simulink library "flexiFlightVis_lib"  (R2018b)
settings: Solver=VariableStepAuto  StartTime=0.0  StopTime=10.0  RelTol=1e-3
values from neighbouring files (symbols this model uses):
  rigid_body = rigidBodyCreate()    [flexiFlightVis_lib_example_init.m]
undefined symbols (not defined in the file or in its folder): config, ffv, ffv_double_array, ffv_double_idx
libraries: dspnetwork x1
settings Model: Creator=yannic  LastModifiedBy=yannic

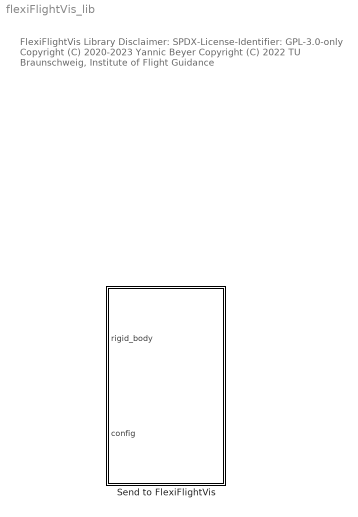
== system flexiFlightVis_lib ==
  note: FlexiFlightVis Library
      |
      | Disclaimer:
      | SPDX-License-Identifier: GPL-3.0-only
      |
      | Copyright (C) 2020-2023 Yannic Beyer
      | Copyright (C) 2022 TU Braunschweig, Institute of Flight Guidance
  Send to FlexiFlightVis : Subsystem  mask{sample_time=1/60, ip_address='localhost', ip_port=4321, wing_cell={}, fuse_cell={}}
      mask prompts: sample_time "sample time"; ip_address "IP address"; ip_port "IP port"; wing_cell "Cell array of wing.state structs"; fuse_cell "Cell array of fuselage.state structs"
      mask init:
      | [ffv,ffv_double_array,ffv_double_idx] = flexiFlightVisBlockInit(gcb,wing_cell,fuse_cell);
      mask DialogControl DescGroupVar Prompt: Send to FlexiFlightVis
      mask DialogControl DescTextVar Prompt: For more information, have a look at the
      mask DialogControl Control2 Prompt: README
      mask DialogControl Control2 Callback: web('https://github.com/iff-gsc/LADAC/tree/main/utilities/interfaces_external_programs/FlexiFlightVis/README.md','-browser')

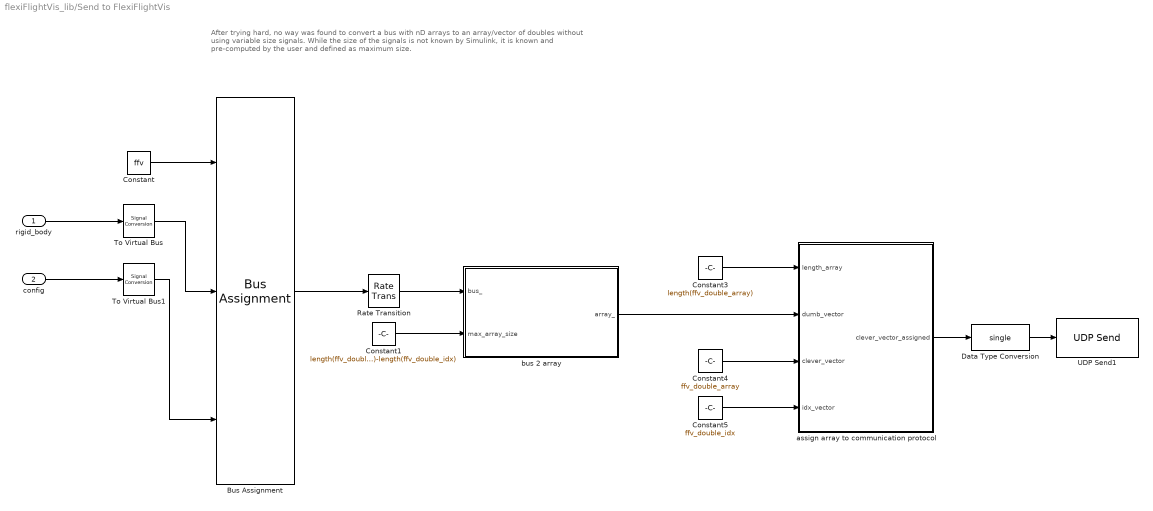
== system flexiFlightVis_lib/Send to FlexiFlightVis ==
  note: After trying hard, no way was found to convert a bus with nD arrays to an array/vector of doubles without using variable size signals.
      | While the size of the signals is not known by Simulink, it is known and pre-computed by the user and defined as maximum size.
  rigid_body : Inport
  config : Inport  Port=2
  Bus Assignment : BusAssignment  AssignedSignals=rigid_body,config
  Constant : Constant  Value=ffv  OutDataTypeStr=Bus: ffv_bus
  Constant1 : Constant  Value=length(ffv_double_array)-length(ffv_double_idx)
  Constant3 : Constant  Value=length(ffv_double_array)
  Constant4 : Constant  Value=ffv_double_array
  Constant5 : Constant  Value=ffv_double_idx
  Data Type Conversion : DataTypeConversion  OutDataTypeStr=single
  Rate Transition : RateTransition  OutPortSampleTime=sample_time
  To Virtual Bus : SignalConversion  ConversionOutput=Virtual bus  OverrideOpt=off
  To Virtual Bus1 : SignalConversion  ConversionOutput=Virtual bus  OverrideOpt=off
  UDP Send1 : dspnetwork/UDP Send  remoteURL=ip_address  remotePort=ip_port  localURL='0.0.0.0'  localPortSource=Automatically determine  localPort=-1  sampletime=-1  blockPlatform=[]  separateLengthPort=0
      settings: SourceProductName=Simulink
  assign array to communication protocol : MATLAB Function  TreatAsAtomicUnit=on
  bus 2 array : MATLAB Function  TreatAsAtomicUnit=on
  wires:
  Constant1/1 -> bus 2 array/2(max_array_size)
  Rate Transition/1 -> bus 2 array/1(bus_)
  assign array to communication protocol/1(clever_vector_assigned) -> Data Type Conversion/1
  Constant3/1 -> assign array to communication protocol/1(length_array)
  Constant4/1 -> assign array to communication protocol/3(clever_vector)
  Constant5/1 -> assign array to communication protocol/4(idx_vector)
  bus 2 array/1(array_) -> assign array to communication protocol/2(dumb_vector)
  Data Type Conversion/1 -> UDP Send1/1
  rigid_body/1 -> To Virtual Bus/1
  Bus Assignment/1 -> Rate Transition/1
  Constant/1 -> Bus Assignment/1
  config/1 -> To Virtual Bus1/1
  To Virtual Bus/1 -> Bus Assignment/2
  To Virtual Bus1/1 -> Bus Assignment/3

== matlab function flexiFlightVis_lib/Send to FlexiFlightVis/assign array to communication protocol ==
  data: length_array input; dumb_vector input size=[1, length(ffv_double_array)-length(ffv_double_idx)]; clever_vector input; idx_vector input; clever_vector_assigned output size=[1, length(ffv_double_array)+1]
function clever_vector_assigned = fcn(length_array, dumb_vector,clever_vector, idx_vector)

clever_vector_row = clever_vector(:)';
idx_vector_row = idx_vector(:)';

clever_out = clever_vector_row;

clever_out(idx_vector_row) = clever_vector_row(idx_vector_row);
% inverse index
idx_2 = setdiff(1:length(clever_out),idx_vector_row);
clever_out(idx_2) = dumb_vector(1:length(idx_2));
clever_vector_assigned = [ length_array, clever_out ];

== matlab function flexiFlightVis_lib/Send to FlexiFlightVis/bus 2 array ==
  data: bus_ input; array_ output size=[1, length(ffv_double_array)-length(ffv_double_idx)]; max_array_size input
function array_ = fcn(bus_,max_array_size)

array_ = bus2array(bus_,max_array_size);
